simulink model "gm_ThreeSines_DrSaher"  (R2018a)
settings: Solver=FixedStepDiscrete  StartTime=0.0  StopTime=0.01  RelTol=1e-3
InitFcn:
  | ST = 2e-8
  | Ts = 2e-8
libraries: hdlmdlgenlib x97, hdlsllib x13, simulink x7, powerlib x1
(part 2 of 3)

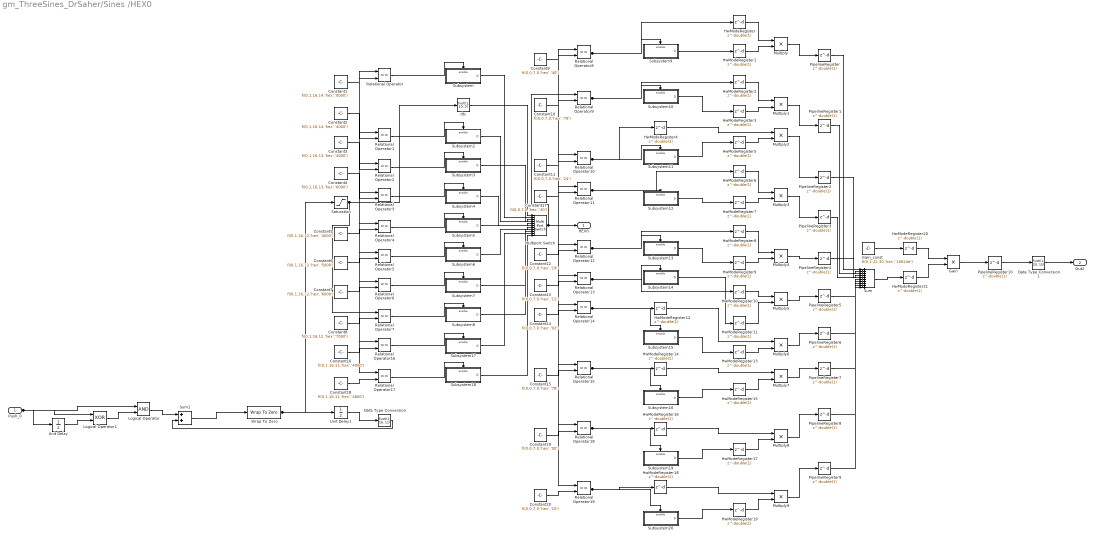
== system gm_ThreeSines_DrSaher/Sines /HEX0 ==
  Push_0 : Inport  PortDimensions=1  SampleTime=2e-08
  Constant1 : Constant  Value=fi(0,1,16,14,'hex','0000')  OutDataTypeStr=fixdt(1, 16, 14)  SampleTime=-1
  Constant10 : Constant  Value=fi(0,0,7,0,'hex','79')  OutDataTypeStr=fixdt(0, 7, 0)  SampleTime=-1
  Constant11 : Constant  Value=fi(0,0,7,0,'hex','24')  OutDataTypeStr=fixdt(0, 7, 0)  SampleTime=-1
  Constant12 : Constant  Value=fi(0,0,7,0,'hex','19')  OutDataTypeStr=fixdt(0, 7, 0)  SampleTime=-1
  Constant13 : Constant  Value=fi(0,0,7,0,'hex','12')  OutDataTypeStr=fixdt(0, 7, 0)  SampleTime=-1
  Constant14 : Constant  Value=fi(0,0,7,0,'hex','02')  OutDataTypeStr=fixdt(0, 7, 0)  SampleTime=-1
  Constant15 : Constant  Value=fi(0,0,7,0,'hex','78')  OutDataTypeStr=fixdt(0, 7, 0)  SampleTime=-1
  Constant16 : Constant  Value=fi(0,1,16,11,'hex','4000')  OutDataTypeStr=fixdt(1, 16, 11)  SampleTime=-1
  Constant17 : Constant  Value=fi(0,0,7,0,'hex','30')  OutDataTypeStr=fixdt(0, 7, 0)  SampleTime=-1
  Constant18 : Constant  Value=fi(0,1,16,11,'hex','4800')  OutDataTypeStr=fixdt(1, 16, 11)  SampleTime=-1
  Constant19 : Constant  Value=fi(0,0,7,0,'hex','00')  OutDataTypeStr=fixdt(0, 7, 0)  SampleTime=-1
  Constant2 : Constant  Value=fi(0,1,16,14,'hex','4000')  OutDataTypeStr=fixdt(1, 16, 14)  SampleTime=-1
  Constant20 : Constant  Value=fi(0,0,7,0,'hex','10')  OutDataTypeStr=fixdt(0, 7, 0)  SampleTime=-1
  Constant3 : Constant  Value=fi(0,1,16,13,'hex','4000')  OutDataTypeStr=fixdt(1, 16, 13)  SampleTime=-1
  Constant4 : Constant  Value=fi(0,1,16,13,'hex','6000')  OutDataTypeStr=fixdt(1, 16, 13)  SampleTime=-1
  Constant5 : Constant  Value=fi(0,1,16,12,'hex','4000')  OutDataTypeStr=fixdt(1, 16, 12)  SampleTime=-1
  Constant6 : Constant  Value=fi(0,1,16,12,'hex','5000')  OutDataTypeStr=fixdt(1, 16, 12)  SampleTime=-1
  Constant7 : Constant  Value=fi(0,1,16,12,'hex','6000')  OutDataTypeStr=fixdt(1, 16, 12)  SampleTime=-1
  Constant8 : Constant  Value=fi(0,1,16,12,'hex','7000')  OutDataTypeStr=fixdt(1, 16, 12)  SampleTime=-1
  Constant9 : Constant  Value=fi(0,0,7,0,'hex','40')  OutDataTypeStr=fixdt(0, 7, 0)  SampleTime=-1
  Data Type Conversion : DataTypeConversion  OutDataTypeStr=fixdt(1, 16, 11)  SampleTime=2e-08
  Data Type Conversion1 : DataTypeConversion  OutDataTypeStr=fixdt(1, 20, 15)  SampleTime=2e-08
  Gain : Product  Inputs=**  OutDataTypeStr=fixdt(1, 44, 44)  SampleTime=2e-08
  Gain_const : Constant  Value=fi(0,1,22,30,'hex','10624e')  OutDataTypeStr=fixdt(1, 22, 30)  SampleTime=-1
  HwModeRegister{,1..21} (22 alike) : Delay  DelayLength=double(1)  InitialCondition=0  InputProcessing=Inherited  SampleTime=2e-08
  Logical Operator : Logic  AllPortsSameDT=off  OutDataTypeStr=boolean  SampleTime=2e-08
  Logical Operator1 : Logic  Operator=XOR  AllPortsSameDT=off  OutDataTypeStr=boolean  SampleTime=2e-08
  Multiply : Product  Inputs=**  OutDataTypeStr=fixdt(1, 16, 10)  SampleTime=2e-08
  Multiply1 : Product  Inputs=**  OutDataTypeStr=fixdt(1, 16, 14)  SampleTime=2e-08
  Multiply2 : Product  Inputs=**  OutDataTypeStr=fixdt(1, 16, 13)  SampleTime=2e-08
  Multiply3 : Product  Inputs=**  OutDataTypeStr=fixdt(1, 16, 13)  SampleTime=2e-08
  Multiply{4..7} (4 alike) : Product  Inputs=**  OutDataTypeStr=fixdt(1, 16, 12)  SampleTime=2e-08
  Multiply8 : Product  Inputs=**  OutDataTypeStr=fixdt(1, 16, 11)  SampleTime=2e-08
  Multiply9 : Product  Inputs=**  OutDataTypeStr=fixdt(1, 16, 11)  SampleTime=2e-08
  Multiport Switch : MultiPortSwitch  DataPortOrder=Zero-based contiguous  Inputs=10  DiagnosticForDefault=None  zeroidx=on  OutDataTypeStr=fixdt(0, 7, 0)  SampleTime=2e-08
  PipelineRegister{,1..10} (11 alike) : Delay  DelayLength=double(1)  InitialCondition=0  InputProcessing=Inherited  SampleTime=2e-08
  Relational Operator{,1..19} (20 alike) : RelationalOperator  Operator===  OutDataTypeStr=boolean  SampleTime=2e-08  RndMeth=Nearest
  Saturation : Saturate  UpperLimit=fi(0,1,21,11,'hex','004800')  LowerLimit=fi(0,1,21,11,'hex','000000')  SampleTime=2e-08  OutDataTypeStr=fixdt(1, 21, 11)
  Subsystem : Subsystem
  Subsystem10 : Subsystem
  Subsystem11 : Subsystem
  Subsystem12 : Subsystem
  Subsystem13 : Subsystem
  Subsystem14 : Subsystem
  Subsystem15 : Subsystem
  Subsystem16 : Subsystem
  Subsystem17 : Subsystem
  Subsystem18 : Subsystem
  Subsystem19 : Subsystem
  Subsystem2 : Subsystem
  Subsystem20 : Subsystem
  Subsystem3 : Subsystem
  Subsystem4 : Subsystem
  Subsystem5 : Subsystem
  Subsystem6 : Subsystem
  Subsystem7 : Subsystem
  Subsystem8 : Subsystem
  Subsystem9 : Subsystem
  Sum : Sum  Inputs=++++++++++  AccumDataTypeStr=fixdt(1, 22, 14)  OutDataTypeStr=fixdt(1, 22, 14)  SampleTime=2e-08
  Sum1 : Sum  AccumDataTypeStr=fixdt(1, 21, 11)  OutDataTypeStr=fixdt(1, 21, 11)  SampleTime=2e-08
  Unit Delay : UnitDelay  SampleTime=2e-08
  Unit Delay1 : UnitDelay  InitialCondition=fi(0,1,21,11,'hex','000000')  SampleTime=2e-08
  Wrap To Zero : simulink/Discontinuities/Wrap To Zero  Threshold=9
      settings: SourceProductName=Simulink  SourceProductBaseCode=SL
  dtc : DataTypeConversion  OutDataTypeStr=fixdt(1, 10, 0)  SampleTime=2e-08
  HEX0 : Outport
  Out2 : Outport  Port=2  OutMax=[0.9]
  wires:
  Constant1/1 -> Relational Operator/2
  Constant10/1 -> Relational Operator9/2
  Constant11/1 -> Relational Operator10/2
  Constant12/1 -> Relational Operator12/2
  Constant13/1 -> Relational Operator13/2
  Constant14/1 -> Relational Operator14/2
  Constant15/1 -> Relational Operator15/2
  Constant16/1 -> Relational Operator16/2
  Constant17/1 -> Relational Operator11/2
  Constant18/1 -> Relational Operator17/2
  Constant19/1 -> Relational Operator18/2
  Constant2/1 -> Relational Operator1/2
  Constant20/1 -> Relational Operator19/2
  Constant3/1 -> Relational Operator2/2
  Constant4/1 -> Relational Operator3/2
  Constant5/1 -> Relational Operator4/2
  Constant6/1 -> Relational Operator5/2
  Constant7/1 -> Relational Operator6/2
  Constant8/1 -> Relational Operator7/2
  Constant9/1 -> Relational Operator8/2
  Data Type Conversion1/1 -> Out2/1
  PipelineRegister10/1 -> Data Type Conversion1/1
  Logical Operator/1 -> Sum1/1
  Logical Operator1/1 -> Logical Operator/2
  PipelineRegister/1 -> Sum/1
  PipelineRegister1/1 -> Sum/2
  PipelineRegister2/1 -> Sum/3
  PipelineRegister3/1 -> Sum/4
  PipelineRegister4/1 -> Sum/5
  PipelineRegister5/1 -> Sum/6
  PipelineRegister6/1 -> Sum/7
  PipelineRegister7/1 -> Sum/8
  PipelineRegister8/1 -> Sum/9
  PipelineRegister9/1 -> Sum/10
  Multiport Switch/1 -> Relational Operator9/1, Relational Operator8/1, Relational Operator19/1, Relational Operator18/1, Relational Operator15/1, Relational Operator14/1, Relational Operator13/1, Relational Operator12/1, Relational Operator11/1, Relational Operator10/1, HEX0/1
  Relational Operator/1 -> Subsystem/Enable
  Relational Operator1/1 -> Subsystem2/Enable
  Relational Operator10/1 -> Subsystem11/Enable, HwModeRegister4/1
  Relational Operator11/1 -> Subsystem12/Enable, HwModeRegister6/1
  Relational Operator12/1 -> Subsystem13/Enable, HwModeRegister8/1
  Relational Operator13/1 -> Subsystem14/Enable, HwModeRegister10/1
  Relational Operator14/1 -> Subsystem15/Enable, HwModeRegister12/1
  Relational Operator15/1 -> Subsystem16/Enable, HwModeRegister14/1
  Relational Operator16/1 -> Subsystem17/Enable
  Relational Operator17/1 -> Subsystem18/Enable
  Relational Operator18/1 -> Subsystem19/Enable, HwModeRegister16/1
  Relational Operator19/1 -> Subsystem20/Enable, HwModeRegister18/1
  Relational Operator2/1 -> Subsystem3/Enable
  Relational Operator3/1 -> Subsystem4/Enable
  Relational Operator4/1 -> Subsystem5/Enable
  Relational Operator5/1 -> Subsystem6/Enable
  Relational Operator6/1 -> Subsystem7/Enable
  Relational Operator7/1 -> Subsystem8/Enable
  Relational Operator8/1 -> Subsystem9/Enable, HwModeRegister/1
  Relational Operator9/1 -> Subsystem10/Enable, HwModeRegister2/1
  Saturation/1 -> Relational Operator7/1, Relational Operator6/1, Relational Operator5/1, Relational Operator4/1, Relational Operator3/1, Relational Operator2/1, Relational Operator17/1, Relational Operator16/1, Relational Operator1/1, Relational Operator/1, dtc/1
  Subsystem/1(0) -> Multiport Switch/2
  Subsystem10/1(0) -> HwModeRegister3/1
  Subsystem11/1(0) -> HwModeRegister5/1
  Subsystem12/1(0) -> HwModeRegister7/1
  Subsystem13/1(0) -> HwModeRegister9/1
  Subsystem14/1(0) -> HwModeRegister11/1
  Subsystem15/1(0) -> HwModeRegister13/1
  Subsystem16/1(0) -> HwModeRegister15/1
  Subsystem17/1(0) -> Multiport Switch/10
  Subsystem18/1(0) -> Multiport Switch/11
  Subsystem19/1(0) -> HwModeRegister17/1
  Subsystem2/1(0) -> Multiport Switch/3
  Subsystem20/1(0) -> HwModeRegister19/1
  Subsystem3/1(0) -> Multiport Switch/4
  Subsystem4/1(0) -> Multiport Switch/5
  Subsystem5/1(0) -> Multiport Switch/6
  Subsystem6/1(0) -> Multiport Switch/7
  Subsystem7/1(0) -> Multiport Switch/8
  Subsystem8/1(0) -> Multiport Switch/9
  Subsystem9/1(0) -> HwModeRegister1/1
  Sum/1 -> HwModeRegister21/1
  Unit Delay/1 -> Logical Operator1/2
  Wrap To Zero/1 -> Saturation/1, Unit Delay1/1
  dtc/1 -> Multiport Switch/1
  Gain_const/1 -> HwModeRegister20/1
  Push_0/1 -> Logical Operator1/1, Logical Operator/1, Unit Delay/1
  Sum1/1 -> Wrap To Zero/1
  Data Type Conversion/1 -> Sum1/2
  Unit Delay1/1 -> Data Type Conversion/1
  Multiply/1 -> PipelineRegister/1
  HwModeRegister/1 -> Multiply/1
  HwModeRegister1/1 -> Multiply/2
  Multiply1/1 -> PipelineRegister1/1
  HwModeRegister2/1 -> Multiply1/1
  HwModeRegister3/1 -> Multiply1/2
  Multiply2/1 -> PipelineRegister2/1
  HwModeRegister4/1 -> Multiply2/1
  HwModeRegister5/1 -> Multiply2/2
  Multiply3/1 -> PipelineRegister3/1
  HwModeRegister6/1 -> Multiply3/1
  HwModeRegister7/1 -> Multiply3/2
  Multiply4/1 -> PipelineRegister4/1
  HwModeRegister8/1 -> Multiply4/1
  HwModeRegister9/1 -> Multiply4/2
  Multiply5/1 -> PipelineRegister5/1
  HwModeRegister10/1 -> Multiply5/1
  HwModeRegister11/1 -> Multiply5/2
  Multiply6/1 -> PipelineRegister6/1
  HwModeRegister12/1 -> Multiply6/1
  HwModeRegister13/1 -> Multiply6/2
  Multiply7/1 -> PipelineRegister7/1
  HwModeRegister14/1 -> Multiply7/1
  HwModeRegister15/1 -> Multiply7/2
  Multiply8/1 -> PipelineRegister8/1
  HwModeRegister16/1 -> Multiply8/1
  HwModeRegister17/1 -> Multiply8/2
  Multiply9/1 -> PipelineRegister9/1
  HwModeRegister18/1 -> Multiply9/1
  HwModeRegister19/1 -> Multiply9/2
  Gain/1 -> PipelineRegister10/1
  HwModeRegister20/1 -> Gain/1
  HwModeRegister21/1 -> Gain/2

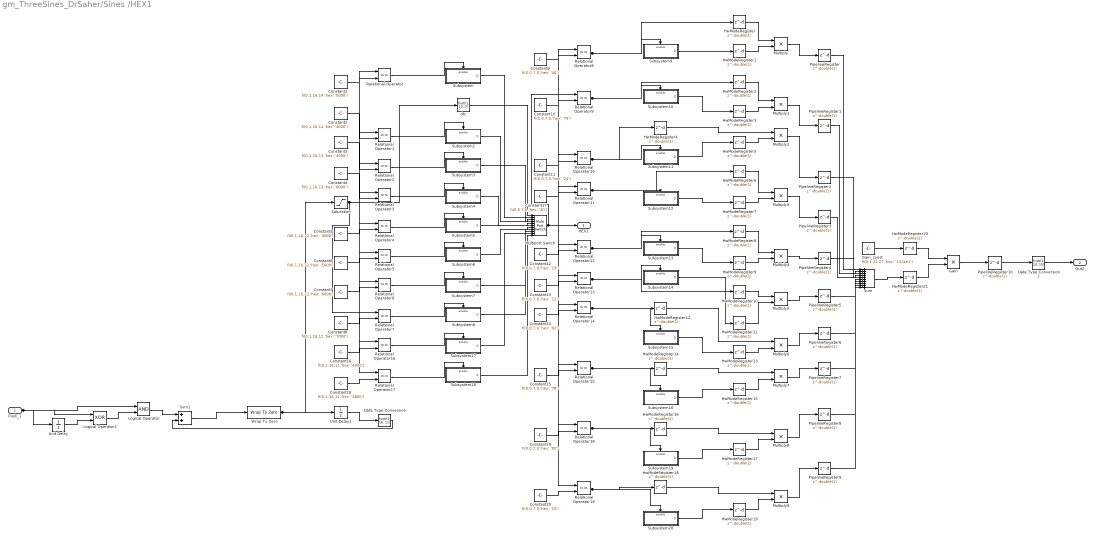
== system gm_ThreeSines_DrSaher/Sines /HEX1 ==
  Push_1 : Inport  PortDimensions=1  SampleTime=2e-08
  Constant1 : Constant  Value=fi(0,1,16,14,'hex','0000')  OutDataTypeStr=fixdt(1, 16, 14)  SampleTime=-1
  Constant10 : Constant  Value=fi(0,0,7,0,'hex','79')  OutDataTypeStr=fixdt(0, 7, 0)  SampleTime=-1
  Constant11 : Constant  Value=fi(0,0,7,0,'hex','24')  OutDataTypeStr=fixdt(0, 7, 0)  SampleTime=-1
  Constant12 : Constant  Value=fi(0,0,7,0,'hex','19')  OutDataTypeStr=fixdt(0, 7, 0)  SampleTime=-1
  Constant13 : Constant  Value=fi(0,0,7,0,'hex','12')  OutDataTypeStr=fixdt(0, 7, 0)  SampleTime=-1
  Constant14 : Constant  Value=fi(0,0,7,0,'hex','02')  OutDataTypeStr=fixdt(0, 7, 0)  SampleTime=-1
  Constant15 : Constant  Value=fi(0,0,7,0,'hex','78')  OutDataTypeStr=fixdt(0, 7, 0)  SampleTime=-1
  Constant16 : Constant  Value=fi(0,1,16,11,'hex','4000')  OutDataTypeStr=fixdt(1, 16, 11)  SampleTime=-1
  Constant17 : Constant  Value=fi(0,0,7,0,'hex','30')  OutDataTypeStr=fixdt(0, 7, 0)  SampleTime=-1
  Constant18 : Constant  Value=fi(0,1,16,11,'hex','4800')  OutDataTypeStr=fixdt(1, 16, 11)  SampleTime=-1
  Constant19 : Constant  Value=fi(0,0,7,0,'hex','00')  OutDataTypeStr=fixdt(0, 7, 0)  SampleTime=-1
  Constant2 : Constant  Value=fi(0,1,16,14,'hex','4000')  OutDataTypeStr=fixdt(1, 16, 14)  SampleTime=-1
  Constant20 : Constant  Value=fi(0,0,7,0,'hex','10')  OutDataTypeStr=fixdt(0, 7, 0)  SampleTime=-1
  Constant3 : Constant  Value=fi(0,1,16,13,'hex','4000')  OutDataTypeStr=fixdt(1, 16, 13)  SampleTime=-1
  Constant4 : Constant  Value=fi(0,1,16,13,'hex','6000')  OutDataTypeStr=fixdt(1, 16, 13)  SampleTime=-1
  Constant5 : Constant  Value=fi(0,1,16,12,'hex','4000')  OutDataTypeStr=fixdt(1, 16, 12)  SampleTime=-1
  Constant6 : Constant  Value=fi(0,1,16,12,'hex','5000')  OutDataTypeStr=fixdt(1, 16, 12)  SampleTime=-1
  Constant7 : Constant  Value=fi(0,1,16,12,'hex','6000')  OutDataTypeStr=fixdt(1, 16, 12)  SampleTime=-1
  Constant8 : Constant  Value=fi(0,1,16,12,'hex','7000')  OutDataTypeStr=fixdt(1, 16, 12)  SampleTime=-1
  Constant9 : Constant  Value=fi(0,0,7,0,'hex','40')  OutDataTypeStr=fixdt(0, 7, 0)  SampleTime=-1
  Data Type Conversion : DataTypeConversion  OutDataTypeStr=fixdt(1, 16, 11)  SampleTime=2e-08
  Data Type Conversion1 : DataTypeConversion  OutDataTypeStr=fixdt(1, 20, 15)  SampleTime=2e-08
  Gain : Product  Inputs=**  OutDataTypeStr=fixdt(1, 44, 41)  SampleTime=2e-08
  Gain_const : Constant  Value=fi(0,1,22,27,'hex','147ae1')  OutDataTypeStr=fixdt(1, 22, 27)  SampleTime=-1
  HwModeRegister{,1..21} (22 alike) : Delay  DelayLength=double(1)  InitialCondition=0  InputProcessing=Inherited  SampleTime=2e-08
  Logical Operator : Logic  AllPortsSameDT=off  OutDataTypeStr=boolean  SampleTime=2e-08
  Logical Operator1 : Logic  Operator=XOR  AllPortsSameDT=off  OutDataTypeStr=boolean  SampleTime=2e-08
  Multiply : Product  Inputs=**  OutDataTypeStr=fixdt(1, 16, 10)  SampleTime=2e-08
  Multiply1 : Product  Inputs=**  OutDataTypeStr=fixdt(1, 16, 14)  SampleTime=2e-08
  Multiply2 : Product  Inputs=**  OutDataTypeStr=fixdt(1, 16, 13)  SampleTime=2e-08
  Multiply3 : Product  Inputs=**  OutDataTypeStr=fixdt(1, 16, 13)  SampleTime=2e-08
  Multiply{4..7} (4 alike) : Product  Inputs=**  OutDataTypeStr=fixdt(1, 16, 12)  SampleTime=2e-08
  Multiply8 : Product  Inputs=**  OutDataTypeStr=fixdt(1, 16, 11)  SampleTime=2e-08
  Multiply9 : Product  Inputs=**  OutDataTypeStr=fixdt(1, 16, 11)  SampleTime=2e-08
  Multiport Switch : MultiPortSwitch  DataPortOrder=Zero-based contiguous  Inputs=10  DiagnosticForDefault=None  zeroidx=on  OutDataTypeStr=fixdt(0, 7, 0)  SampleTime=2e-08
  PipelineRegister{,1..10} (11 alike) : Delay  DelayLength=double(1)  InitialCondition=0  InputProcessing=Inherited  SampleTime=2e-08
  Relational Operator{,1..19} (20 alike) : RelationalOperator  Operator===  OutDataTypeStr=boolean  SampleTime=2e-08  RndMeth=Nearest
  Saturation : Saturate  UpperLimit=fi(0,1,21,11,'hex','004800')  LowerLimit=fi(0,1,21,11,'hex','000000')  SampleTime=2e-08  OutDataTypeStr=fixdt(1, 21, 11)
  Subsystem : Subsystem
  Subsystem10 : Subsystem
  Subsystem11 : Subsystem
  Subsystem12 : Subsystem
  Subsystem13 : Subsystem
  Subsystem14 : Subsystem
  Subsystem15 : Subsystem
  Subsystem16 : Subsystem
  Subsystem17 : Subsystem
  Subsystem18 : Subsystem
  Subsystem19 : Subsystem
  Subsystem2 : Subsystem
  Subsystem20 : Subsystem
  Subsystem3 : Subsystem
  Subsystem4 : Subsystem
  Subsystem5 : Subsystem
  Subsystem6 : Subsystem
  Subsystem7 : Subsystem
  Subsystem8 : Subsystem
  Subsystem9 : Subsystem
  Sum : Sum  Inputs=++++++++++  AccumDataTypeStr=fixdt(1, 22, 14)  OutDataTypeStr=fixdt(1, 22, 14)  SampleTime=2e-08
  Sum1 : Sum  AccumDataTypeStr=fixdt(1, 21, 11)  OutDataTypeStr=fixdt(1, 21, 11)  SampleTime=2e-08
  Unit Delay : UnitDelay  SampleTime=2e-08
  Unit Delay1 : UnitDelay  InitialCondition=fi(0,1,21,11,'hex','000000')  SampleTime=2e-08
  Wrap To Zero : simulink/Discontinuities/Wrap To Zero  Threshold=9
      settings: SourceProductName=Simulink  SourceProductBaseCode=SL
  dtc : DataTypeConversion  OutDataTypeStr=fixdt(1, 10, 0)  SampleTime=2e-08
  HEX1 : Outport
  Out2 : Outport  Port=2  OutMax=[0.9]
  wires:
  Constant1/1 -> Relational Operator/2
  Constant10/1 -> Relational Operator9/2
  Constant11/1 -> Relational Operator10/2
  Constant12/1 -> Relational Operator12/2
  Constant13/1 -> Relational Operator13/2
  Constant14/1 -> Relational Operator14/2
  Constant15/1 -> Relational Operator15/2
  Constant16/1 -> Relational Operator16/2
  Constant17/1 -> Relational Operator11/2
  Constant18/1 -> Relational Operator17/2
  Constant19/1 -> Relational Operator18/2
  Constant2/1 -> Relational Operator1/2
  Constant20/1 -> Relational Operator19/2
  Constant3/1 -> Relational Operator2/2
  Constant4/1 -> Relational Operator3/2
  Constant5/1 -> Relational Operator4/2
  Constant6/1 -> Relational Operator5/2
  Constant7/1 -> Relational Operator6/2
  Constant8/1 -> Relational Operator7/2
  Constant9/1 -> Relational Operator8/2
  Data Type Conversion1/1 -> Out2/1
  PipelineRegister10/1 -> Data Type Conversion1/1
  Logical Operator/1 -> Sum1/1
  Logical Operator1/1 -> Logical Operator/2
  PipelineRegister/1 -> Sum/1
  PipelineRegister1/1 -> Sum/2
  PipelineRegister2/1 -> Sum/3
  PipelineRegister3/1 -> Sum/4
  PipelineRegister4/1 -> Sum/5
  PipelineRegister5/1 -> Sum/6
  PipelineRegister6/1 -> Sum/7
  PipelineRegister7/1 -> Sum/8
  PipelineRegister8/1 -> Sum/9
  PipelineRegister9/1 -> Sum/10
  Multiport Switch/1 -> Relational Operator9/1, Relational Operator8/1, Relational Operator19/1, Relational Operator18/1, Relational Operator15/1, Relational Operator14/1, Relational Operator13/1, Relational Operator12/1, Relational Operator11/1, Relational Operator10/1, HEX1/1
  Relational Operator/1 -> Subsystem/Enable
  Relational Operator1/1 -> Subsystem2/Enable
  Relational Operator10/1 -> Subsystem11/Enable, HwModeRegister4/1
  Relational Operator11/1 -> Subsystem12/Enable, HwModeRegister6/1
  Relational Operator12/1 -> Subsystem13/Enable, HwModeRegister8/1
  Relational Operator13/1 -> Subsystem14/Enable, HwModeRegister10/1
  Relational Operator14/1 -> Subsystem15/Enable, HwModeRegister12/1
  Relational Operator15/1 -> Subsystem16/Enable, HwModeRegister14/1
  Relational Operator16/1 -> Subsystem17/Enable
  Relational Operator17/1 -> Subsystem18/Enable
  Relational Operator18/1 -> Subsystem19/Enable, HwModeRegister16/1
  Relational Operator19/1 -> Subsystem20/Enable, HwModeRegister18/1
  Relational Operator2/1 -> Subsystem3/Enable
  Relational Operator3/1 -> Subsystem4/Enable
  Relational Operator4/1 -> Subsystem5/Enable
  Relational Operator5/1 -> Subsystem6/Enable
  Relational Operator6/1 -> Subsystem7/Enable
  Relational Operator7/1 -> Subsystem8/Enable
  Relational Operator8/1 -> Subsystem9/Enable, HwModeRegister/1
  Relational Operator9/1 -> Subsystem10/Enable, HwModeRegister2/1
  Saturation/1 -> Relational Operator7/1, Relational Operator6/1, Relational Operator5/1, Relational Operator4/1, Relational Operator3/1, Relational Operator2/1, Relational Operator17/1, Relational Operator16/1, Relational Operator1/1, Relational Operator/1, dtc/1
  Subsystem/1(0) -> Multiport Switch/2
  Subsystem10/1(0) -> HwModeRegister3/1
  Subsystem11/1(0) -> HwModeRegister5/1
  Subsystem12/1(0) -> HwModeRegister7/1
  Subsystem13/1(0) -> HwModeRegister9/1
  Subsystem14/1(0) -> HwModeRegister11/1
  Subsystem15/1(0) -> HwModeRegister13/1
  Subsystem16/1(0) -> HwModeRegister15/1
  Subsystem17/1(0) -> Multiport Switch/10
  Subsystem18/1(0) -> Multiport Switch/11
  Subsystem19/1(0) -> HwModeRegister17/1
  Subsystem2/1(0) -> Multiport Switch/3
  Subsystem20/1(0) -> HwModeRegister19/1
  Subsystem3/1(0) -> Multiport Switch/4
  Subsystem4/1(0) -> Multiport Switch/5
  Subsystem5/1(0) -> Multiport Switch/6
  Subsystem6/1(0) -> Multiport Switch/7
  Subsystem7/1(0) -> Multiport Switch/8
  Subsystem8/1(0) -> Multiport Switch/9
  Subsystem9/1(0) -> HwModeRegister1/1
  Sum/1 -> HwModeRegister21/1
  Unit Delay/1 -> Logical Operator1/2
  Wrap To Zero/1 -> Saturation/1, Unit Delay1/1
  dtc/1 -> Multiport Switch/1
  Gain_const/1 -> HwModeRegister20/1
  Push_1/1 -> Logical Operator1/1, Logical Operator/1, Unit Delay/1
  Sum1/1 -> Wrap To Zero/1
  Data Type Conversion/1 -> Sum1/2
  Unit Delay1/1 -> Data Type Conversion/1
  Multiply/1 -> PipelineRegister/1
  HwModeRegister/1 -> Multiply/1
  HwModeRegister1/1 -> Multiply/2
  Multiply1/1 -> PipelineRegister1/1
  HwModeRegister2/1 -> Multiply1/1
  HwModeRegister3/1 -> Multiply1/2
  Multiply2/1 -> PipelineRegister2/1
  HwModeRegister4/1 -> Multiply2/1
  HwModeRegister5/1 -> Multiply2/2
  Multiply3/1 -> PipelineRegister3/1
  HwModeRegister6/1 -> Multiply3/1
  HwModeRegister7/1 -> Multiply3/2
  Multiply4/1 -> PipelineRegister4/1
  HwModeRegister8/1 -> Multiply4/1
  HwModeRegister9/1 -> Multiply4/2
  Multiply5/1 -> PipelineRegister5/1
  HwModeRegister10/1 -> Multiply5/1
  HwModeRegister11/1 -> Multiply5/2
  Multiply6/1 -> PipelineRegister6/1
  HwModeRegister12/1 -> Multiply6/1
  HwModeRegister13/1 -> Multiply6/2
  Multiply7/1 -> PipelineRegister7/1
  HwModeRegister14/1 -> Multiply7/1
  HwModeRegister15/1 -> Multiply7/2
  Multiply8/1 -> PipelineRegister8/1
  HwModeRegister16/1 -> Multiply8/1
  HwModeRegister17/1 -> Multiply8/2
  Multiply9/1 -> PipelineRegister9/1
  HwModeRegister18/1 -> Multiply9/1
  HwModeRegister19/1 -> Multiply9/2
  Gain/1 -> PipelineRegister10/1
  HwModeRegister20/1 -> Gain/1
  HwModeRegister21/1 -> Gain/2

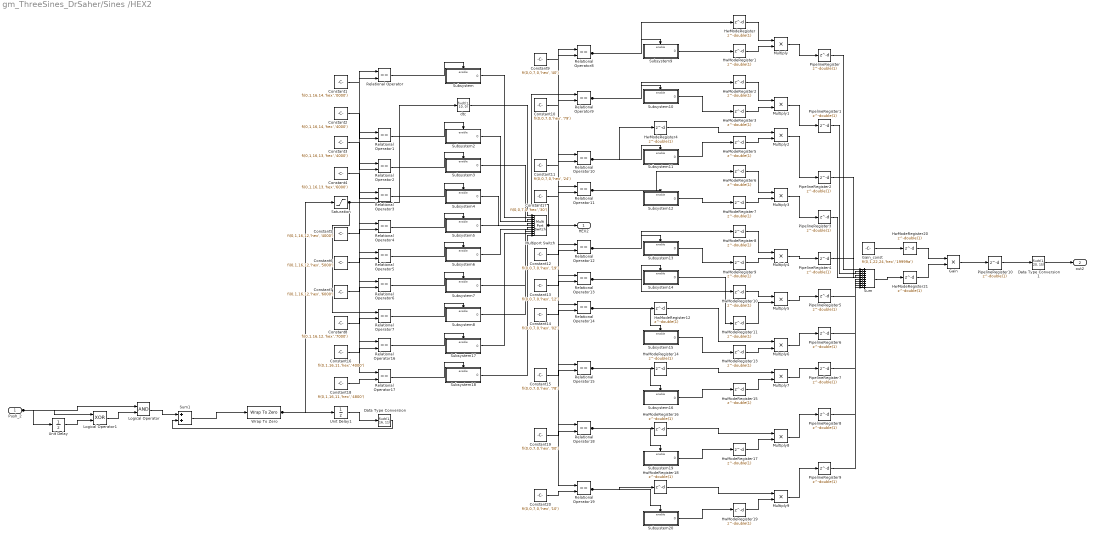
== system gm_ThreeSines_DrSaher/Sines /HEX2 ==
  Push_2 : Inport  PortDimensions=1  SampleTime=2e-08
  Constant1 : Constant  Value=fi(0,1,16,14,'hex','0000')  OutDataTypeStr=fixdt(1, 16, 14)  SampleTime=-1
  Constant10 : Constant  Value=fi(0,0,7,0,'hex','79')  OutDataTypeStr=fixdt(0, 7, 0)  SampleTime=-1
  Constant11 : Constant  Value=fi(0,0,7,0,'hex','24')  OutDataTypeStr=fixdt(0, 7, 0)  SampleTime=-1
  Constant12 : Constant  Value=fi(0,0,7,0,'hex','19')  OutDataTypeStr=fixdt(0, 7, 0)  SampleTime=-1
  Constant13 : Constant  Value=fi(0,0,7,0,'hex','12')  OutDataTypeStr=fixdt(0, 7, 0)  SampleTime=-1
  Constant14 : Constant  Value=fi(0,0,7,0,'hex','02')  OutDataTypeStr=fixdt(0, 7, 0)  SampleTime=-1
  Constant15 : Constant  Value=fi(0,0,7,0,'hex','78')  OutDataTypeStr=fixdt(0, 7, 0)  SampleTime=-1
  Constant16 : Constant  Value=fi(0,1,16,11,'hex','4000')  OutDataTypeStr=fixdt(1, 16, 11)  SampleTime=-1
  Constant17 : Constant  Value=fi(0,0,7,0,'hex','30')  OutDataTypeStr=fixdt(0, 7, 0)  SampleTime=-1
  Constant18 : Constant  Value=fi(0,1,16,11,'hex','4800')  OutDataTypeStr=fixdt(1, 16, 11)  SampleTime=-1
  Constant19 : Constant  Value=fi(0,0,7,0,'hex','00')  OutDataTypeStr=fixdt(0, 7, 0)  SampleTime=-1
  Constant2 : Constant  Value=fi(0,1,16,14,'hex','4000')  OutDataTypeStr=fixdt(1, 16, 14)  SampleTime=-1
  Constant20 : Constant  Value=fi(0,0,7,0,'hex','10')  OutDataTypeStr=fixdt(0, 7, 0)  SampleTime=-1
  Constant3 : Constant  Value=fi(0,1,16,13,'hex','4000')  OutDataTypeStr=fixdt(1, 16, 13)  SampleTime=-1
  Constant4 : Constant  Value=fi(0,1,16,13,'hex','6000')  OutDataTypeStr=fixdt(1, 16, 13)  SampleTime=-1
  Constant5 : Constant  Value=fi(0,1,16,12,'hex','4000')  OutDataTypeStr=fixdt(1, 16, 12)  SampleTime=-1
  Constant6 : Constant  Value=fi(0,1,16,12,'hex','5000')  OutDataTypeStr=fixdt(1, 16, 12)  SampleTime=-1
  Constant7 : Constant  Value=fi(0,1,16,12,'hex','6000')  OutDataTypeStr=fixdt(1, 16, 12)  SampleTime=-1
  Constant8 : Constant  Value=fi(0,1,16,12,'hex','7000')  OutDataTypeStr=fixdt(1, 16, 12)  SampleTime=-1
  Constant9 : Constant  Value=fi(0,0,7,0,'hex','40')  OutDataTypeStr=fixdt(0, 7, 0)  SampleTime=-1
  Data Type Conversion : DataTypeConversion  OutDataTypeStr=fixdt(1, 16, 11)  SampleTime=2e-08
  Data Type Conversion1 : DataTypeConversion  OutDataTypeStr=fixdt(1, 20, 15)  SampleTime=2e-08
  Gain : Product  Inputs=**  OutDataTypeStr=fixdt(1, 44, 38)  SampleTime=2e-08
  Gain_const : Constant  Value=fi(0,1,22,24,'hex','19999a')  OutDataTypeStr=fixdt(1, 22, 24)  SampleTime=-1
  HwModeRegister{,1..21} (22 alike) : Delay  DelayLength=double(1)  InitialCondition=0  InputProcessing=Inherited  SampleTime=2e-08
  Logical Operator : Logic  AllPortsSameDT=off  OutDataTypeStr=boolean  SampleTime=2e-08
  Logical Operator1 : Logic  Operator=XOR  AllPortsSameDT=off  OutDataTypeStr=boolean  SampleTime=2e-08
  Multiply : Product  Inputs=**  OutDataTypeStr=fixdt(1, 16, 10)  SampleTime=2e-08
  Multiply1 : Product  Inputs=**  OutDataTypeStr=fixdt(1, 16, 14)  SampleTime=2e-08
  Multiply2 : Product  Inputs=**  OutDataTypeStr=fixdt(1, 16, 13)  SampleTime=2e-08
  Multiply3 : Product  Inputs=**  OutDataTypeStr=fixdt(1, 16, 13)  SampleTime=2e-08
  Multiply{4..7} (4 alike) : Product  Inputs=**  OutDataTypeStr=fixdt(1, 16, 12)  SampleTime=2e-08
  Multiply8 : Product  Inputs=**  OutDataTypeStr=fixdt(1, 16, 11)  SampleTime=2e-08
  Multiply9 : Product  Inputs=**  OutDataTypeStr=fixdt(1, 16, 11)  SampleTime=2e-08
  Multiport Switch : MultiPortSwitch  DataPortOrder=Zero-based contiguous  Inputs=10  DiagnosticForDefault=None  zeroidx=on  OutDataTypeStr=fixdt(0, 7, 0)  SampleTime=2e-08
  PipelineRegister{,1..10} (11 alike) : Delay  DelayLength=double(1)  InitialCondition=0  InputProcessing=Inherited  SampleTime=2e-08
  Relational Operator{,1..19} (20 alike) : RelationalOperator  Operator===  OutDataTypeStr=boolean  SampleTime=2e-08  RndMeth=Nearest
  Saturation : Saturate  UpperLimit=fi(0,1,21,11,'hex','004800')  LowerLimit=fi(0,1,21,11,'hex','000000')  SampleTime=2e-08  OutDataTypeStr=fixdt(1, 21, 11)
  Subsystem : Subsystem
  Subsystem10 : Subsystem
  Subsystem11 : Subsystem
  Subsystem12 : Subsystem
  Subsystem13 : Subsystem
  Subsystem14 : Subsystem
  Subsystem15 : Subsystem
  Subsystem16 : Subsystem
  Subsystem17 : Subsystem
  Subsystem18 : Subsystem
  Subsystem19 : Subsystem
  Subsystem2 : Subsystem
  Subsystem20 : Subsystem
  Subsystem3 : Subsystem
  Subsystem4 : Subsystem
  Subsystem5 : Subsystem
  Subsystem6 : Subsystem
  Subsystem7 : Subsystem
  Subsystem8 : Subsystem
  Subsystem9 : Subsystem
  Sum : Sum  Inputs=++++++++++  AccumDataTypeStr=fixdt(1, 22, 14)  OutDataTypeStr=fixdt(1, 22, 14)  SampleTime=2e-08
  Sum1 : Sum  AccumDataTypeStr=fixdt(1, 21, 11)  OutDataTypeStr=fixdt(1, 21, 11)  SampleTime=2e-08
  Unit Delay : UnitDelay  SampleTime=2e-08
  Unit Delay1 : UnitDelay  InitialCondition=fi(0,1,21,11,'hex','000000')  SampleTime=2e-08
  Wrap To Zero : simulink/Discontinuities/Wrap To Zero  Threshold=9
      settings: SourceProductName=Simulink  SourceProductBaseCode=SL
  dtc : DataTypeConversion  OutDataTypeStr=fixdt(1, 10, 0)  SampleTime=2e-08
  HEX2 : Outport
  out2 : Outport  Port=2  OutMax=[0.9]
  wires:
  Constant1/1 -> Relational Operator/2
  Constant10/1 -> Relational Operator9/2
  Constant11/1 -> Relational Operator10/2
  Constant12/1 -> Relational Operator12/2
  Constant13/1 -> Relational Operator13/2
  Constant14/1 -> Relational Operator14/2
  Constant15/1 -> Relational Operator15/2
  Constant16/1 -> Relational Operator16/2
  Constant17/1 -> Relational Operator11/2
  Constant18/1 -> Relational Operator17/2
  Constant19/1 -> Relational Operator18/2
  Constant2/1 -> Relational Operator1/2
  Constant20/1 -> Relational Operator19/2
  Constant3/1 -> Relational Operator2/2
  Constant4/1 -> Relational Operator3/2
  Constant5/1 -> Relational Operator4/2
  Constant6/1 -> Relational Operator5/2
  Constant7/1 -> Relational Operator6/2
  Constant8/1 -> Relational Operator7/2
  Constant9/1 -> Relational Operator8/2
  Data Type Conversion1/1 -> out2/1
  PipelineRegister10/1 -> Data Type Conversion1/1
  Logical Operator/1 -> Sum1/1
  Logical Operator1/1 -> Logical Operator/2
  PipelineRegister/1 -> Sum/1
  PipelineRegister1/1 -> Sum/2
  PipelineRegister2/1 -> Sum/3
  PipelineRegister3/1 -> Sum/4
  PipelineRegister4/1 -> Sum/5
  PipelineRegister5/1 -> Sum/6
  PipelineRegister6/1 -> Sum/7
  PipelineRegister7/1 -> Sum/8
  PipelineRegister8/1 -> Sum/9
  PipelineRegister9/1 -> Sum/10
  Multiport Switch/1 -> Relational Operator9/1, Relational Operator8/1, Relational Operator19/1, Relational Operator18/1, Relational Operator15/1, Relational Operator14/1, Relational Operator13/1, Relational Operator12/1, Relational Operator11/1, Relational Operator10/1, HEX2/1
  Relational Operator/1 -> Subsystem/Enable
  Relational Operator1/1 -> Subsystem2/Enable
  Relational Operator10/1 -> Subsystem11/Enable, HwModeRegister4/1
  Relational Operator11/1 -> Subsystem12/Enable, HwModeRegister6/1
  Relational Operator12/1 -> Subsystem13/Enable, HwModeRegister8/1
  Relational Operator13/1 -> Subsystem14/Enable, HwModeRegister10/1
  Relational Operator14/1 -> Subsystem15/Enable, HwModeRegister12/1
  Relational Operator15/1 -> Subsystem16/Enable, HwModeRegister14/1
  Relational Operator16/1 -> Subsystem17/Enable
  Relational Operator17/1 -> Subsystem18/Enable
  Relational Operator18/1 -> Subsystem19/Enable, HwModeRegister16/1
  Relational Operator19/1 -> Subsystem20/Enable, HwModeRegister18/1
  Relational Operator2/1 -> Subsystem3/Enable
  Relational Operator3/1 -> Subsystem4/Enable
  Relational Operator4/1 -> Subsystem5/Enable
  Relational Operator5/1 -> Subsystem6/Enable
  Relational Operator6/1 -> Subsystem7/Enable
  Relational Operator7/1 -> Subsystem8/Enable
  Relational Operator8/1 -> Subsystem9/Enable, HwModeRegister/1
  Relational Operator9/1 -> Subsystem10/Enable, HwModeRegister2/1
  Saturation/1 -> Relational Operator7/1, Relational Operator6/1, Relational Operator5/1, Relational Operator4/1, Relational Operator3/1, Relational Operator2/1, Relational Operator17/1, Relational Operator16/1, Relational Operator1/1, Relational Operator/1, dtc/1
  Subsystem/1(0) -> Multiport Switch/2
  Subsystem10/1(0) -> HwModeRegister3/1
  Subsystem11/1(0) -> HwModeRegister5/1
  Subsystem12/1(0) -> HwModeRegister7/1
  Subsystem13/1(0) -> HwModeRegister9/1
  Subsystem14/1(0) -> HwModeRegister11/1
  Subsystem15/1(0) -> HwModeRegister13/1
  Subsystem16/1(0) -> HwModeRegister15/1
  Subsystem17/1(0) -> Multiport Switch/10
  Subsystem18/1(0) -> Multiport Switch/11
  Subsystem19/1(0) -> HwModeRegister17/1
  Subsystem2/1(0) -> Multiport Switch/3
  Subsystem20/1(0) -> HwModeRegister19/1
  Subsystem3/1(0) -> Multiport Switch/4
  Subsystem4/1(0) -> Multiport Switch/5
  Subsystem5/1(0) -> Multiport Switch/6
  Subsystem6/1(0) -> Multiport Switch/7
  Subsystem7/1(0) -> Multiport Switch/8
  Subsystem8/1(0) -> Multiport Switch/9
  Subsystem9/1(0) -> HwModeRegister1/1
  Sum/1 -> HwModeRegister21/1
  Unit Delay/1 -> Logical Operator1/2
  Wrap To Zero/1 -> Saturation/1, Unit Delay1/1
  dtc/1 -> Multiport Switch/1
  Gain_const/1 -> HwModeRegister20/1
  Push_2/1 -> Logical Operator1/1, Logical Operator/1, Unit Delay/1
  Sum1/1 -> Wrap To Zero/1
  Data Type Conversion/1 -> Sum1/2
  Unit Delay1/1 -> Data Type Conversion/1
  Multiply/1 -> PipelineRegister/1
  HwModeRegister/1 -> Multiply/1
  HwModeRegister1/1 -> Multiply/2
  Multiply1/1 -> PipelineRegister1/1
  HwModeRegister2/1 -> Multiply1/1
  HwModeRegister3/1 -> Multiply1/2
  Multiply2/1 -> PipelineRegister2/1
  HwModeRegister4/1 -> Multiply2/1
  HwModeRegister5/1 -> Multiply2/2
  Multiply3/1 -> PipelineRegister3/1
  HwModeRegister6/1 -> Multiply3/1
  HwModeRegister7/1 -> Multiply3/2
  Multiply4/1 -> PipelineRegister4/1
  HwModeRegister8/1 -> Multiply4/1
  HwModeRegister9/1 -> Multiply4/2
  Multiply5/1 -> PipelineRegister5/1
  HwModeRegister10/1 -> Multiply5/1
  HwModeRegister11/1 -> Multiply5/2
  Multiply6/1 -> PipelineRegister6/1
  HwModeRegister12/1 -> Multiply6/1
  HwModeRegister13/1 -> Multiply6/2
  Multiply7/1 -> PipelineRegister7/1
  HwModeRegister14/1 -> Multiply7/1
  HwModeRegister15/1 -> Multiply7/2
  Multiply8/1 -> PipelineRegister8/1
  HwModeRegister16/1 -> Multiply8/1
  HwModeRegister17/1 -> Multiply8/2
  Multiply9/1 -> PipelineRegister9/1
  HwModeRegister18/1 -> Multiply9/1
  HwModeRegister19/1 -> Multiply9/2
  Gain/1 -> PipelineRegister10/1
  HwModeRegister20/1 -> Gain/1
  HwModeRegister21/1 -> Gain/2

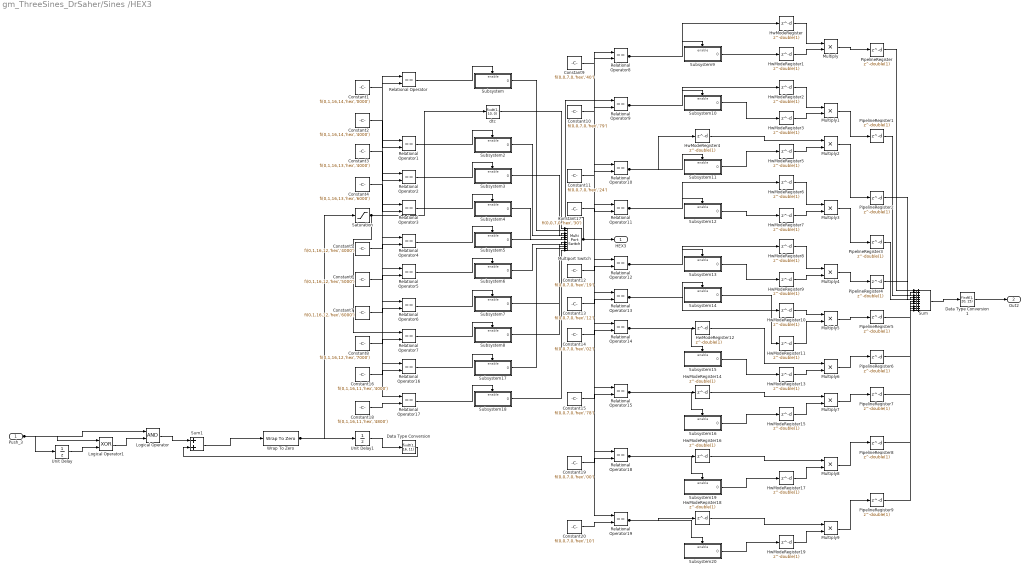
== system gm_ThreeSines_DrSaher/Sines /HEX3 ==
  Push_3 : Inport  PortDimensions=1  SampleTime=2e-08
  Constant1 : Constant  Value=fi(0,1,16,14,'hex','0000')  OutDataTypeStr=fixdt(1, 16, 14)  SampleTime=-1
  Constant10 : Constant  Value=fi(0,0,7,0,'hex','79')  OutDataTypeStr=fixdt(0, 7, 0)  SampleTime=-1
  Constant11 : Constant  Value=fi(0,0,7,0,'hex','24')  OutDataTypeStr=fixdt(0, 7, 0)  SampleTime=-1
  Constant12 : Constant  Value=fi(0,0,7,0,'hex','19')  OutDataTypeStr=fixdt(0, 7, 0)  SampleTime=-1
  Constant13 : Constant  Value=fi(0,0,7,0,'hex','12')  OutDataTypeStr=fixdt(0, 7, 0)  SampleTime=-1
  Constant14 : Constant  Value=fi(0,0,7,0,'hex','02')  OutDataTypeStr=fixdt(0, 7, 0)  SampleTime=-1
  Constant15 : Constant  Value=fi(0,0,7,0,'hex','78')  OutDataTypeStr=fixdt(0, 7, 0)  SampleTime=-1
  Constant16 : Constant  Value=fi(0,1,16,11,'hex','4000')  OutDataTypeStr=fixdt(1, 16, 11)  SampleTime=-1
  Constant17 : Constant  Value=fi(0,0,7,0,'hex','30')  OutDataTypeStr=fixdt(0, 7, 0)  SampleTime=-1
  Constant18 : Constant  Value=fi(0,1,16,11,'hex','4800')  OutDataTypeStr=fixdt(1, 16, 11)  SampleTime=-1
  Constant19 : Constant  Value=fi(0,0,7,0,'hex','00')  OutDataTypeStr=fixdt(0, 7, 0)  SampleTime=-1
  Constant2 : Constant  Value=fi(0,1,16,14,'hex','4000')  OutDataTypeStr=fixdt(1, 16, 14)  SampleTime=-1
  Constant20 : Constant  Value=fi(0,0,7,0,'hex','10')  OutDataTypeStr=fixdt(0, 7, 0)  SampleTime=-1
  Constant3 : Constant  Value=fi(0,1,16,13,'hex','4000')  OutDataTypeStr=fixdt(1, 16, 13)  SampleTime=-1
  Constant4 : Constant  Value=fi(0,1,16,13,'hex','6000')  OutDataTypeStr=fixdt(1, 16, 13)  SampleTime=-1
  Constant5 : Constant  Value=fi(0,1,16,12,'hex','4000')  OutDataTypeStr=fixdt(1, 16, 12)  SampleTime=-1
  Constant6 : Constant  Value=fi(0,1,16,12,'hex','5000')  OutDataTypeStr=fixdt(1, 16, 12)  SampleTime=-1
  Constant7 : Constant  Value=fi(0,1,16,12,'hex','6000')  OutDataTypeStr=fixdt(1, 16, 12)  SampleTime=-1
  Constant8 : Constant  Value=fi(0,1,16,12,'hex','7000')  OutDataTypeStr=fixdt(1, 16, 12)  SampleTime=-1
  Constant9 : Constant  Value=fi(0,0,7,0,'hex','40')  OutDataTypeStr=fixdt(0, 7, 0)  SampleTime=-1
  Data Type Conversion : DataTypeConversion  OutDataTypeStr=fixdt(1, 16, 11)  SampleTime=2e-08
  Data Type Conversion1 : DataTypeConversion  OutDataTypeStr=fixdt(1, 20, 15)  SampleTime=2e-08
  HwModeRegister{,1..19} (20 alike) : Delay  DelayLength=double(1)  InitialCondition=0  InputProcessing=Inherited  SampleTime=2e-08
  Logical Operator : Logic  AllPortsSameDT=off  OutDataTypeStr=boolean  SampleTime=2e-08
  Logical Operator1 : Logic  Operator=XOR  AllPortsSameDT=off  OutDataTypeStr=boolean  SampleTime=2e-08
  Multiply : Product  Inputs=**  OutDataTypeStr=fixdt(1, 16, 10)  SampleTime=2e-08
  Multiply1 : Product  Inputs=**  OutDataTypeStr=fixdt(1, 16, 14)  SampleTime=2e-08
  Multiply2 : Product  Inputs=**  OutDataTypeStr=fixdt(1, 16, 13)  SampleTime=2e-08
  Multiply3 : Product  Inputs=**  OutDataTypeStr=fixdt(1, 16, 13)  SampleTime=2e-08
  Multiply{4..7} (4 alike) : Product  Inputs=**  OutDataTypeStr=fixdt(1, 16, 12)  SampleTime=2e-08
  Multiply8 : Product  Inputs=**  OutDataTypeStr=fixdt(1, 16, 11)  SampleTime=2e-08
  Multiply9 : Product  Inputs=**  OutDataTypeStr=fixdt(1, 16, 11)  SampleTime=2e-08
  Multiport Switch : MultiPortSwitch  DataPortOrder=Zero-based contiguous  Inputs=10  DiagnosticForDefault=None  zeroidx=on  OutDataTypeStr=fixdt(0, 7, 0)  SampleTime=2e-08
  PipelineRegister{,1..9} (10 alike) : Delay  DelayLength=double(1)  InitialCondition=0  InputProcessing=Inherited  SampleTime=2e-08
  Relational Operator{,1..19} (20 alike) : RelationalOperator  Operator===  OutDataTypeStr=boolean  SampleTime=2e-08  RndMeth=Nearest
  Saturation : Saturate  UpperLimit=fi(0,1,21,11,'hex','004800')  LowerLimit=fi(0,1,21,11,'hex','000000')  SampleTime=2e-08  OutDataTypeStr=fixdt(1, 21, 11)
  Subsystem : Subsystem
  Subsystem10 : Subsystem
  Subsystem11 : Subsystem
  Subsystem12 : Subsystem
  Subsystem13 : Subsystem
  Subsystem14 : Subsystem
  Subsystem15 : Subsystem
  Subsystem16 : Subsystem
  Subsystem17 : Subsystem
  Subsystem18 : Subsystem
  Subsystem19 : Subsystem
  Subsystem2 : Subsystem
  Subsystem20 : Subsystem
  Subsystem3 : Subsystem
  Subsystem4 : Subsystem
  Subsystem5 : Subsystem
  Subsystem6 : Subsystem
  Subsystem7 : Subsystem
  Subsystem8 : Subsystem
  Subsystem9 : Subsystem
  Sum : Sum  Inputs=++++++++++  AccumDataTypeStr=fixdt(1, 22, 14)  OutDataTypeStr=fixdt(1, 22, 14)  SampleTime=2e-08
  Sum1 : Sum  AccumDataTypeStr=fixdt(1, 21, 11)  OutDataTypeStr=fixdt(1, 21, 11)  SampleTime=2e-08
  Unit Delay : UnitDelay  SampleTime=2e-08
  Unit Delay1 : UnitDelay  InitialCondition=fi(0,1,21,11,'hex','000000')  SampleTime=2e-08
  Wrap To Zero : simulink/Discontinuities/Wrap To Zero  Threshold=9
      settings: SourceProductName=Simulink  SourceProductBaseCode=SL
  dtc : DataTypeConversion  OutDataTypeStr=fixdt(1, 10, 0)  SampleTime=2e-08
  HEX3 : Outport
  Out2 : Outport  Port=2  OutMax=[0.9]
  wires:
  Constant1/1 -> Relational Operator/2
  Constant10/1 -> Relational Operator9/2
  Constant11/1 -> Relational Operator10/2
  Constant12/1 -> Relational Operator12/2
  Constant13/1 -> Relational Operator13/2
  Constant14/1 -> Relational Operator14/2
  Constant15/1 -> Relational Operator15/2
  Constant16/1 -> Relational Operator16/2
  Constant17/1 -> Relational Operator11/2
  Constant18/1 -> Relational Operator17/2
  Constant19/1 -> Relational Operator18/2
  Constant2/1 -> Relational Operator1/2
  Constant20/1 -> Relational Operator19/2
  Constant3/1 -> Relational Operator2/2
  Constant4/1 -> Relational Operator3/2
  Constant5/1 -> Relational Operator4/2
  Constant6/1 -> Relational Operator5/2
  Constant7/1 -> Relational Operator6/2
  Constant8/1 -> Relational Operator7/2
  Constant9/1 -> Relational Operator8/2
  Data Type Conversion1/1 -> Out2/1
  Logical Operator/1 -> Sum1/1
  Logical Operator1/1 -> Logical Operator/2
  PipelineRegister/1 -> Sum/1
  PipelineRegister1/1 -> Sum/2
  PipelineRegister2/1 -> Sum/3
  PipelineRegister3/1 -> Sum/4
  PipelineRegister4/1 -> Sum/5
  PipelineRegister5/1 -> Sum/6
  PipelineRegister6/1 -> Sum/7
  PipelineRegister7/1 -> Sum/8
  PipelineRegister8/1 -> Sum/9
  PipelineRegister9/1 -> Sum/10
  Multiport Switch/1 -> Relational Operator9/1, Relational Operator8/1, Relational Operator19/1, Relational Operator18/1, Relational Operator15/1, Relational Operator14/1, Relational Operator13/1, Relational Operator12/1, Relational Operator11/1, Relational Operator10/1, HEX3/1
  Relational Operator/1 -> Subsystem/Enable
  Relational Operator1/1 -> Subsystem2/Enable
  Relational Operator10/1 -> Subsystem11/Enable, HwModeRegister4/1
  Relational Operator11/1 -> Subsystem12/Enable, HwModeRegister6/1
  Relational Operator12/1 -> Subsystem13/Enable, HwModeRegister8/1
  Relational Operator13/1 -> Subsystem14/Enable, HwModeRegister10/1
  Relational Operator14/1 -> Subsystem15/Enable, HwModeRegister12/1
  Relational Operator15/1 -> Subsystem16/Enable, HwModeRegister14/1
  Relational Operator16/1 -> Subsystem17/Enable
  Relational Operator17/1 -> Subsystem18/Enable
  Relational Operator18/1 -> Subsystem19/Enable, HwModeRegister16/1
  Relational Operator19/1 -> Subsystem20/Enable, HwModeRegister18/1
  Relational Operator2/1 -> Subsystem3/Enable
  Relational Operator3/1 -> Subsystem4/Enable
  Relational Operator4/1 -> Subsystem5/Enable
  Relational Operator5/1 -> Subsystem6/Enable
  Relational Operator6/1 -> Subsystem7/Enable
  Relational Operator7/1 -> Subsystem8/Enable
  Relational Operator8/1 -> Subsystem9/Enable, HwModeRegister/1
  Relational Operator9/1 -> Subsystem10/Enable, HwModeRegister2/1
  Saturation/1 -> Relational Operator7/1, Relational Operator6/1, Relational Operator5/1, Relational Operator4/1, Relational Operator3/1, Relational Operator2/1, Relational Operator17/1, Relational Operator16/1, Relational Operator1/1, Relational Operator/1, dtc/1
  Subsystem/1(0) -> Multiport Switch/2
  Subsystem10/1(0) -> HwModeRegister3/1
  Subsystem11/1(0) -> HwModeRegister5/1
  Subsystem12/1(0) -> HwModeRegister7/1
  Subsystem13/1(0) -> HwModeRegister9/1
  Subsystem14/1(0) -> HwModeRegister11/1
  Subsystem15/1(0) -> HwModeRegister13/1
  Subsystem16/1(0) -> HwModeRegister15/1
  Subsystem17/1(0) -> Multiport Switch/10
  Subsystem18/1(0) -> Multiport Switch/11
  Subsystem19/1(0) -> HwModeRegister17/1
  Subsystem2/1(0) -> Multiport Switch/3
  Subsystem20/1(0) -> HwModeRegister19/1
  Subsystem3/1(0) -> Multiport Switch/4
  Subsystem4/1(0) -> Multiport Switch/5
  Subsystem5/1(0) -> Multiport Switch/6
  Subsystem6/1(0) -> Multiport Switch/7
  Subsystem7/1(0) -> Multiport Switch/8
  Subsystem8/1(0) -> Multiport Switch/9
  Subsystem9/1(0) -> HwModeRegister1/1
  Sum/1 -> Data Type Conversion1/1
  Unit Delay/1 -> Logical Operator1/2
  Wrap To Zero/1 -> Saturation/1, Unit Delay1/1
  dtc/1 -> Multiport Switch/1
  Push_3/1 -> Logical Operator1/1, Logical Operator/1, Unit Delay/1
  Sum1/1 -> Wrap To Zero/1
  Data Type Conversion/1 -> Sum1/2
  Unit Delay1/1 -> Data Type Conversion/1
  Multiply/1 -> PipelineRegister/1
  HwModeRegister/1 -> Multiply/1
  HwModeRegister1/1 -> Multiply/2
  Multiply1/1 -> PipelineRegister1/1
  HwModeRegister2/1 -> Multiply1/1
  HwModeRegister3/1 -> Multiply1/2
  Multiply2/1 -> PipelineRegister2/1
  HwModeRegister4/1 -> Multiply2/1
  HwModeRegister5/1 -> Multiply2/2
  Multiply3/1 -> PipelineRegister3/1
  HwModeRegister6/1 -> Multiply3/1
  HwModeRegister7/1 -> Multiply3/2
  Multiply4/1 -> PipelineRegister4/1
  HwModeRegister8/1 -> Multiply4/1
  HwModeRegister9/1 -> Multiply4/2
  Multiply5/1 -> PipelineRegister5/1
  HwModeRegister10/1 -> Multiply5/1
  HwModeRegister11/1 -> Multiply5/2
  Multiply6/1 -> PipelineRegister6/1
  HwModeRegister12/1 -> Multiply6/1
  HwModeRegister13/1 -> Multiply6/2
  Multiply7/1 -> PipelineRegister7/1
  HwModeRegister14/1 -> Multiply7/1
  HwModeRegister15/1 -> Multiply7/2
  Multiply8/1 -> PipelineRegister8/1
  HwModeRegister16/1 -> Multiply8/1
  HwModeRegister17/1 -> Multiply8/2
  Multiply9/1 -> PipelineRegister9/1
  HwModeRegister18/1 -> Multiply9/1
  HwModeRegister19/1 -> Multiply9/2

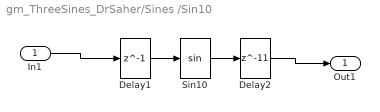
== system gm_ThreeSines_DrSaher/Sines /Sin10 ==
  In1 : Inport
  Delay1 : Delay  DelayLength=1  InputProcessing=Inherited
  Delay2 : Delay  DelayLength=11  InputProcessing=Inherited
  Sin10 : Trigonometry  ApproximationMethod=CORDIC
  Out1 : Outport
  wires:
  In1/1 -> Delay1/1
  Delay1/1 -> Sin10/1
  Sin10/1 -> Delay2/1
  Delay2/1 -> Out1/1

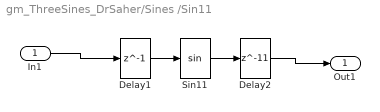
== system gm_ThreeSines_DrSaher/Sines /Sin11 ==
  In1 : Inport
  Delay1 : Delay  DelayLength=1  InputProcessing=Inherited
  Delay2 : Delay  DelayLength=11  InputProcessing=Inherited
  Sin11 : Trigonometry  ApproximationMethod=CORDIC
  Out1 : Outport
  wires:
  In1/1 -> Delay1/1
  Delay1/1 -> Sin11/1
  Sin11/1 -> Delay2/1
  Delay2/1 -> Out1/1

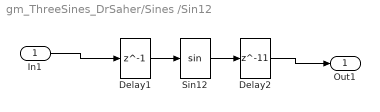
== system gm_ThreeSines_DrSaher/Sines /Sin12 ==
  In1 : Inport
  Delay1 : Delay  DelayLength=1  InputProcessing=Inherited
  Delay2 : Delay  DelayLength=11  InputProcessing=Inherited
  Sin12 : Trigonometry  ApproximationMethod=CORDIC
  Out1 : Outport
  wires:
  In1/1 -> Delay1/1
  Delay1/1 -> Sin12/1
  Sin12/1 -> Delay2/1
  Delay2/1 -> Out1/1

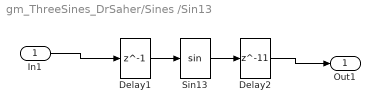
== system gm_ThreeSines_DrSaher/Sines /Sin13 ==
  In1 : Inport
  Delay1 : Delay  DelayLength=1  InputProcessing=Inherited
  Delay2 : Delay  DelayLength=11  InputProcessing=Inherited
  Sin13 : Trigonometry  ApproximationMethod=CORDIC
  Out1 : Outport
  wires:
  In1/1 -> Delay1/1
  Delay1/1 -> Sin13/1
  Sin13/1 -> Delay2/1
  Delay2/1 -> Out1/1

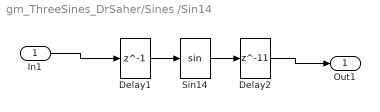
== system gm_ThreeSines_DrSaher/Sines /Sin14 ==
  In1 : Inport
  Delay1 : Delay  DelayLength=1  InputProcessing=Inherited
  Delay2 : Delay  DelayLength=11  InputProcessing=Inherited
  Sin14 : Trigonometry  ApproximationMethod=CORDIC
  Out1 : Outport
  wires:
  In1/1 -> Delay1/1
  Delay1/1 -> Sin14/1
  Sin14/1 -> Delay2/1
  Delay2/1 -> Out1/1

== system gm_ThreeSines_DrSaher/Sines /Sin15 ==
  In1 : Inport
  Delay1 : Delay  DelayLength=1  InputProcessing=Inherited
  Delay2 : Delay  DelayLength=11  InputProcessing=Inherited
  Sin15 : Trigonometry  ApproximationMethod=CORDIC
  Out1 : Outport
  wires:
  In1/1 -> Delay1/1
  Delay1/1 -> Sin15/1
  Sin15/1 -> Delay2/1
  Delay2/1 -> Out1/1

== system gm_ThreeSines_DrSaher/Sines /Sin4 ==
  In1 : Inport
  Delay1 : Delay  DelayLength=1  InputProcessing=Inherited
  Delay2 : Delay  DelayLength=11  InputProcessing=Inherited
  Sin4 : Trigonometry  ApproximationMethod=CORDIC
  Out1 : Outport
  wires:
  In1/1 -> Delay1/1
  Delay1/1 -> Sin4/1
  Sin4/1 -> Delay2/1
  Delay2/1 -> Out1/1

== system gm_ThreeSines_DrSaher/Sines /Sin5 ==
  In1 : Inport
  Delay1 : Delay  DelayLength=1  InputProcessing=Inherited
  Delay2 : Delay  DelayLength=11  InputProcessing=Inherited
  Sin5 : Trigonometry  ApproximationMethod=CORDIC
  Out1 : Outport
  wires:
  In1/1 -> Delay1/1
  Delay1/1 -> Sin5/1
  Sin5/1 -> Delay2/1
  Delay2/1 -> Out1/1

== system gm_ThreeSines_DrSaher/Sines /Sin6 ==
  In1 : Inport
  Delay1 : Delay  DelayLength=1  InputProcessing=Inherited
  Delay2 : Delay  DelayLength=11  InputProcessing=Inherited
  Sin6 : Trigonometry  ApproximationMethod=CORDIC
  Out1 : Outport
  wires:
  In1/1 -> Delay1/1
  Delay1/1 -> Sin6/1
  Sin6/1 -> Delay2/1
  Delay2/1 -> Out1/1

== system gm_ThreeSines_DrSaher/Sines /Sin7 ==
  In1 : Inport
  Delay1 : Delay  DelayLength=1  InputProcessing=Inherited
  Delay2 : Delay  DelayLength=11  InputProcessing=Inherited
  Sin7 : Trigonometry  ApproximationMethod=CORDIC
  Out1 : Outport
  wires:
  In1/1 -> Delay1/1
  Delay1/1 -> Sin7/1
  Sin7/1 -> Delay2/1
  Delay2/1 -> Out1/1

== system gm_ThreeSines_DrSaher/Sines /Sin8 ==
  In1 : Inport
  Delay1 : Delay  DelayLength=1  InputProcessing=Inherited
  Delay2 : Delay  DelayLength=11  InputProcessing=Inherited
  Sin8 : Trigonometry  ApproximationMethod=CORDIC
  Out1 : Outport
  wires:
  In1/1 -> Delay1/1
  Delay1/1 -> Sin8/1
  Sin8/1 -> Delay2/1
  Delay2/1 -> Out1/1

== system gm_ThreeSines_DrSaher/Sines /Sin9 ==
  In1 : Inport
  Delay1 : Delay  DelayLength=1  InputProcessing=Inherited
  Delay2 : Delay  DelayLength=11  InputProcessing=Inherited
  Sin9 : Trigonometry  ApproximationMethod=CORDIC
  Out1 : Outport
  wires:
  In1/1 -> Delay1/1
  Delay1/1 -> Sin9/1
  Sin9/1 -> Delay2/1
  Delay2/1 -> Out1/1

== system gm_ThreeSines_DrSaher/Sines /Subsystem ==
  In1 : Inport  PortDimensions=1  SampleTime=2e-08
  Enable : EnablePort
  Out1 : Outport  InitialOutput=0
  wires:
  In1/1 -> Out1/1

== system gm_ThreeSines_DrSaher/Sines /Subsystem1 ==
  In1 : Inport  PortDimensions=1  SampleTime=2e-08
  Enable : EnablePort
  Out1 : Outport  InitialOutput=0
  wires:
  In1/1 -> Out1/1

== system gm_ThreeSines_DrSaher/Sines /Subsystem10 ==
  In1 : Inport  PortDimensions=1  SampleTime=2e-08
  Enable : EnablePort
  Out1 : Outport  InitialOutput=0
  wires:
  In1/1 -> Out1/1

== system gm_ThreeSines_DrSaher/Sines /Subsystem11 ==
  In1 : Inport  PortDimensions=1  SampleTime=2e-08
  Enable : EnablePort
  Out1 : Outport  InitialOutput=0
  wires:
  In1/1 -> Out1/1

== system gm_ThreeSines_DrSaher/Sines /Subsystem12 ==
  In1 : Inport  PortDimensions=1  SampleTime=2e-08
  Enable : EnablePort
  Out1 : Outport  InitialOutput=0
  wires:
  In1/1 -> Out1/1

== system gm_ThreeSines_DrSaher/Sines /Subsystem13 ==
  In1 : Inport  PortDimensions=1  SampleTime=2e-08
  Enable : EnablePort
  Out1 : Outport  InitialOutput=0
  wires:
  In1/1 -> Out1/1

== system gm_ThreeSines_DrSaher/Sines /Subsystem2 ==
  In1 : Inport  PortDimensions=1  SampleTime=2e-08
  Enable : EnablePort
  Out1 : Outport  InitialOutput=0
  wires:
  In1/1 -> Out1/1

== system gm_ThreeSines_DrSaher/Sines /Subsystem3 ==
  In1 : Inport  PortDimensions=1  SampleTime=2e-08
  Enable : EnablePort
  Out1 : Outport  InitialOutput=0
  wires:
  In1/1 -> Out1/1

== system gm_ThreeSines_DrSaher/Sines /Subsystem4 ==
  In1 : Inport  PortDimensions=1  SampleTime=2e-08
  Enable : EnablePort
  Out1 : Outport  InitialOutput=0
  wires:
  In1/1 -> Out1/1

== system gm_ThreeSines_DrSaher/Sines /Subsystem5 ==
  In1 : Inport  PortDimensions=1  SampleTime=2e-08
  Enable : EnablePort
  Out1 : Outport  InitialOutput=0
  wires:
  In1/1 -> Out1/1

== system gm_ThreeSines_DrSaher/Sines /Subsystem6 ==
  In1 : Inport  PortDimensions=1  SampleTime=2e-08
  Enable : EnablePort
  Out1 : Outport  InitialOutput=0
  wires:
  In1/1 -> Out1/1

== system gm_ThreeSines_DrSaher/Sines /Subsystem7 ==
  In1 : Inport  PortDimensions=1  SampleTime=2e-08
  Enable : EnablePort
  Out1 : Outport  InitialOutput=0
  wires:
  In1/1 -> Out1/1

== system gm_ThreeSines_DrSaher/Sines /Subsystem8 ==
  In1 : Inport  PortDimensions=1  SampleTime=2e-08
  Enable : EnablePort
  Out1 : Outport  InitialOutput=0
  wires:
  In1/1 -> Out1/1

== system gm_ThreeSines_DrSaher/Sines /Subsystem9 ==
  In1 : Inport  PortDimensions=1  SampleTime=2e-08
  Enable : EnablePort
  Out1 : Outport  InitialOutput=0
  wires:
  In1/1 -> Out1/1

== system gm_ThreeSines_DrSaher/Sines /aPA_Save ==
  MulNumber : Inport  PortDimensions=1  SampleTime=2e-08
  Enable : EnablePort
  MulResult : Outport  InitialOutput=0
  wires:
  MulNumber/1 -> MulResult/1

== system gm_ThreeSines_DrSaher/Sines /aPB_Save ==
  MulNumber : Inport  PortDimensions=1  SampleTime=2e-08
  Enable : EnablePort
  MulResult : Outport  InitialOutput=0
  wires:
  MulNumber/1 -> MulResult/1

== system gm_ThreeSines_DrSaher/Sines /aPC_Save ==
  MulNumber : Inport  PortDimensions=1  SampleTime=2e-08
  Enable : EnablePort
  MulResult : Outport  InitialOutput=0
  wires:
  MulNumber/1 -> MulResult/1

== system gm_ThreeSines_DrSaher/Sines /bPA_Save ==
  MulNumber : Inport  PortDimensions=1  SampleTime=2e-08
  Enable : EnablePort
  MulResult : Outport  InitialOutput=0
  wires:
  MulNumber/1 -> MulResult/1

== system gm_ThreeSines_DrSaher/Sines /bPB_Save ==
  MulNumber : Inport  PortDimensions=1  SampleTime=2e-08
  Enable : EnablePort
  MulResult : Outport  InitialOutput=0
  wires:
  MulNumber/1 -> MulResult/1

== system gm_ThreeSines_DrSaher/Sines /bPC_Save ==
  MulNumber : Inport  PortDimensions=1  SampleTime=2e-08
  Enable : EnablePort
  MulResult : Outport  InitialOutput=0
  wires:
  MulNumber/1 -> MulResult/1
